simulink model "sldemo_radar"  (Simulink 7.6)
settings: Solver=ode5  SolverMode=SingleTasking  StartTime=0.0  StopTime=100  FixedStep=0.1  MaxStep=0.1  RelTol=1e-3  AbsTol=1e-6
StartFcn:
  | clear radarLogsOut
StopFcn:
  | aero_radplot;
model workspace (MATLAB code in the model file):
  | g = 32.2;    % Acceleration due to gravity (ft/sec^2)
  | tauc = 5;    % Correlation time of aircraft cross axis acceleration
  | tauT = 4;    % Correlation time of aircraft thrust axis acceleration
  | Speed = 400; % Initial speed of aircraft in y direction feet/sec
  | deltat = 1;  % Radar update rate (also hard-coded in extkalman.m)
libraries: simulink x2
Description:
  | Radar tracking Model
  | 
  | This demonstration shows how to use an extended Kalman filter to estimate an
  | aircraft's position from radar measurements. The filter implementation is found
  | in the file aero_extkalman.m.  The vehicle model is vectorized so that all
  | 3 degrees of freedom are computed using one set of blocks.
  | 
  | At the end of the simulation, a figure displays the following information:
  | 
  | * The actual trajectory compared to the estimated trajectory
  | * The estimation residual for range
  | * The actual, measured, and estimated position
CloseFcn:
  | h=findobj('type','figure');if ~isempty(h);close(h);end
  | clear radarLogsOut
settings Model: Creator=The MathWorks Inc.  CovMetricSettings=d  ExtModeTrigMode=oneshot  ExtModeArmWhenConnect=off  ExtModeAutoUpdateStatusClock=off
settings DataIOCC: LimitDataPoints=off  SaveOutput=off  SaveTime=off  TimeSaveName=t_sim  SignalLoggingName=radarLogsOut
settings OptimizationCC: InlineParams=on  InlineInvariantSignals=on  StateBitsets=on  DataBitsets=on  UseTempVars=on  ZeroExternalMemoryAtStartup=off  ZeroInternalMemoryAtStartup=off  NoFixptDivByZeroProtection=on  OptimizeModelRefInitCode=on  LifeSpan=1  BufferReusableBoundary=off
settings DebuggingCC: SaveWithParameterizedLinksMsg=none  CheckExecutionContextPreStartOutputMsg=on  CheckExecutionContextRuntimeOutputMsg=on  SignalResolutionControl=TryResolveAllWithWarning  SolverPrmCheckMsg=none  MultiTaskDSMMsg=warning  MultiTaskCondExecSysMsg=none
settings SFSimCC: SimParseCustomCode=off
settings RTWCC: SystemTargetFile=ert.tlc  TLCOptions=-p0 -aWarnNonSaturatedBlocks=0  TemplateMakefile=ert_default_tmf  Description=RTW Embedded Coder (no auto configuration)  GenerateReport=on  RTWVerbose=off  ProcessScript=ert_make_rtw_hook  IncludeHyperlinkInReport=on  LaunchReport=on  IncludeERTFirstTime=on
settings CodeAppCC: ForceParamTrailComments=on  IgnoreCustomStorageClasses=off  SimulinkDataObjDesc=on  CustomSymbolStrGlobalVar=rt$N$M  CustomSymbolStrType=$N$M  CustomSymbolStrFcn=$N$M$F  CustomSymbolStrMacro=$N$M  InsertBlockDesc=on
settings ERTTargetCC: TargetFcnLib=ansi_tfl_tmw.mat  MultiwordLength=2048  GenerateSampleERTMain=on  IncludeMdlTerminateFcn=off  SupportComplex=off  SupportContinuousTime=on  SupportNonInlinedSFcns=on  InlinedParameterPlacement=NonHierarchical  ERTCustomFileTemplate=example_file_process.tlc  ConvertIfToSwitch=off

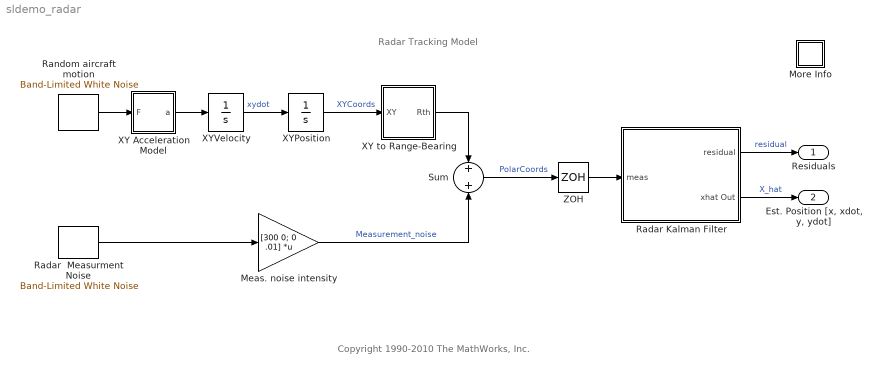
== system sldemo_radar ==
  note: Radar Tracking Model
  note: Copyright 1990-2010 The MathWorks, Inc.
  Meas. noise intensity : Gain  Gain=[300 0; 0 .01]  Multiplication=Matrix(K*u) (u vector)
  More Info : Subsystem
      settings: OpenFcn=showdemo(bdroot(gcb))
      mask Display: disp('?')
  Radar Kalman Filter : Subsystem  TreatAsAtomicUnit=on
  Radar  Measurment Noise : simulink/Sources/Band-Limited White Noise  SystemSampleTime=-1  Cov=[1 1]  Ts=0.1  seed=[52341 62341]
  Random aircraft motion : simulink/Sources/Band-Limited White Noise  SystemSampleTime=-1  Cov=[0.001 .001]  Ts=0.1  seed=[58413 74925]
  Sum : Sum  Inputs=2  SaturateOnIntegerOverflow=on  InputSameDT=on  OutDataTypeStr=Inherit: Same as first input
  XY Acceleration Model : Subsystem
  XY to Range-Bearing : Subsystem
      mask Type: xy2rtheta
      mask Description:
      | Vector transformation from cartesian to polar coordinates.
      | input:   [x, y]
      | output: [r, theta]
      | 
      | r = hypot(x,y));
      | theta = atan2(y,x);
      mask Help: Use "Look under mask" to see the implementation, done in Simulink blocks.
      mask Display: plot(0,0,100,100,[24,20,15,20,20],[85,95,85,95,20],[80,20,95,85,95,85],[70,20,20,15,20,24],[56,56,55,52,50,46],[20,26,31,35,38,42])
  XYPosition : Integrator
  XYVelocity : Integrator  InitialCondition=[0, Speed]
  ZOH : ZeroOrderHold  SampleTime=deltat
  Residuals : Outport
  "Est. Position [x, xdot, y, ydot]" : Outport  Port=2
  wires:
  XYPosition/1 -> XY to Range-Bearing/1(XY)  "XYCoords"
  XY to Range-Bearing/1(Rth) -> Sum/1
  Sum/1 -> ZOH/1  "PolarCoords"
  XYVelocity/1 -> XYPosition/1  "xydot"
  XY Acceleration Model/1(a) -> XYVelocity/1
  Radar Kalman Filter/1(residual) -> Residuals/1  "residual"
  Random aircraft motion/1 -> XY Acceleration Model/1(F)
  Radar Kalman Filter/2(xhat Out) -> "Est. Position [x, xdot, y, ydot]"/1  "X_hat"
  Radar  Measurment Noise/1 -> Meas. noise intensity/1
  Meas. noise intensity/1 -> Sum/2  "Measurement_noise"
  ZOH/1 -> Radar Kalman Filter/1(meas)

== system sldemo_radar/More Info ==

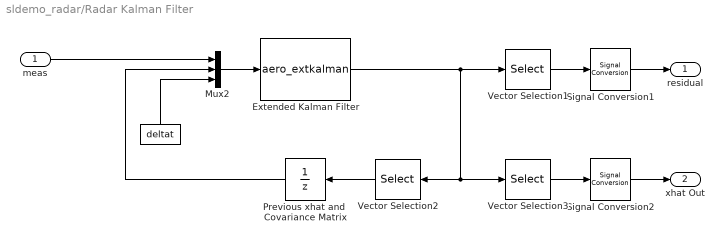
== system sldemo_radar/Radar Kalman Filter ==
  meas : Inport
  " " : Constant  Value=deltat
  Extended Kalman Filter : MATLABFcn  MATLABFcn=aero_extkalman  OutputDimensions=23
  Mux2 : Mux  Inputs=3
  Previous xhat and  Covariance Matrix : UnitDelay  X0=[0.001; 0.01; 0.001; 400; zeros(16,1)]  SampleTime=deltat
  Signal Conversion1 : SignalConversion  ConversionOutput=Contiguous copy  OverrideOpt=on
  Signal Conversion2 : SignalConversion  ConversionOutput=Contiguous copy  OverrideOpt=on
  Vector Selection1 : Selector  InputPortWidth=23  IndexOptions=Index vector (dialog)  Indices=[1,2]  OutputSizes=1
      settings: AttributesFormatString=elts = %<Elements>
  Vector Selection2 : Selector  InputPortWidth=23  IndexOptions=Index vector (dialog)  Indices=[3:22]  OutputSizes=1
      settings: AttributesFormatString=elts = %<Elements>
  Vector Selection3 : Selector  InputPortWidth=23  IndexOptions=Index vector (dialog)  Indices=[3,4,5,6]  OutputSizes=1
      settings: AttributesFormatString=elts = %<Elements>
  residual : Outport  InitialOutput=0
  xhat Out : Outport  Port=2  InitialOutput=0
  wires:
  Vector Selection1/1 -> Signal Conversion1/1
  Mux2/1 -> Extended Kalman Filter/1
  Previous xhat and  Covariance Matrix/1 -> Mux2/2
  " "/1 -> Mux2/3
  Vector Selection3/1 -> Signal Conversion2/1
  Extended Kalman Filter/1 -> Vector Selection3/1, Vector Selection2/1, Vector Selection1/1
  meas/1 -> Mux2/1
  Vector Selection2/1 -> Previous xhat and  Covariance Matrix/1
  Signal Conversion1/1 -> residual/1
  Signal Conversion2/1 -> xhat Out/1

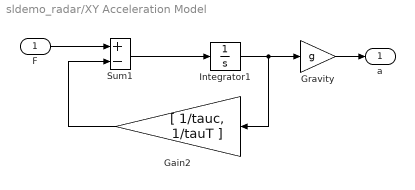
== system sldemo_radar/XY Acceleration Model ==
  F : Inport
  Gain2 : Gain  Gain=[ 1/tauc, 1/tauT ]  SaturateOnIntegerOverflow=on  OutDataTypeStr=Inherit: Same as input  ParamDataTypeStr=Inherit: Same as input
  Gravity : Gain  Gain=g  SaturateOnIntegerOverflow=on  OutDataTypeStr=Inherit: Same as input  ParamDataTypeStr=Inherit: Same as input
  Integrator1 : Integrator
  Sum1 : Sum  Inputs=+-  SaturateOnIntegerOverflow=on  InputSameDT=on  OutDataTypeStr=Inherit: Same as first input
  a : Outport  InitialOutput=0
  wires:
  F/1 -> Sum1/1
  Gain2/1 -> Sum1/2
  Integrator1/1 -> Gravity/1, Gain2/1
  Sum1/1 -> Integrator1/1
  Gravity/1 -> a/1

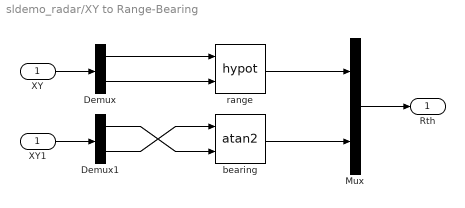
== system sldemo_radar/XY to Range-Bearing ==
  XY : Inport
  Demux : Demux  Outputs=2
  Demux1 : Demux  Outputs=2
  Mux : Mux  Inputs=2
  XY1 : InportShadow  Port=1
  bearing : Trigonometry  Operator=atan2
  range : Math  Operator=hypot  SaturateOnIntegerOverflow=on
  Rth : Outport  InitialOutput=0
  wires:
  Mux/1 -> Rth/1
  range/1 -> Mux/1
  XY/1 -> Demux/1
  Demux/1 -> range/1
  Demux/2 -> range/2
  XY1/1 -> Demux1/1
  bearing/1 -> Mux/2
  Demux1/1 -> bearing/2
  Demux1/2 -> bearing/1
